simulink model "chapter5_2"  (R2018b)
settings: Solver=VariableStepAuto  StartTime=0.0  StopTime=10.0  RelTol=1e-3
settings Model: Creator=nharada  LastModifiedBy=nharada

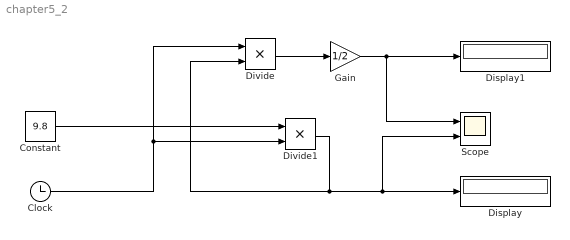
== system chapter5_2 ==
  Clock : Clock
  Constant : Constant  Value=9.8
  Display : Display
  Display1 : Display
  Divide : Product  Inputs=**
  Divide1 : Product  Inputs=**
  Gain : Gain  Gain=1/2
  Scope : Scope  NumInputPorts=2
  wires:
  Constant/1 -> Divide1/1
  Clock/1 -> Divide/1, Divide1/2
  Divide/1 -> Gain/1
  Gain/1 -> Scope/1, Display1/1
  Divide1/1 -> Divide/2, Scope/2, Display/1
